simulink model "hexsim_block_model"  (R2015b)
settings: Solver=ode45  StartTime=0.0  StopTime=inf  FixedStep=0.002  RelTol=1e-3
InitFcn:
  | param
values from neighbouring files (symbols this model uses):
  colors = lines(length(row))    [adaptive_coefficients_figure.m]    (also in drawAircraft.m = [edgecolor; edgecolor; edgecolor; edgecolor; footprintcolor])
  V = V*R    [drawAircraft.m]
undefined symbols (not defined in the file or in its folder): attitude_controller, drawAircraft, F, P, position_controller
libraries: simulink x4
settings Model: Creator=beard  LastModifiedBy=magiccjae
settings DataIOCC: SaveFormat=Array  SignalLoggingSaveFormat=ModelDataLogs
settings OptimizationCC: ExpressionDepthLimit=2147483647  InitFltsAndDblsToZero=on
settings DebuggingCC: UnderspecifiedInitializationDetection=Classic  MergeDetectMultiDrivingBlocksExec=none  SolverPrmCheckMsg=warning  FcnCallInpInsideContextMsg=UseLocalSettings  StateNameClashWarn=warning
settings HardwareCC: ProdBitPerPointer=32  ProdLargestAtomicFloat=None  ProdIntDivRoundTo=Undefined  ProdEndianess=Unspecified  ProdWordSize=32  ProdHWDeviceType=32-bit Generic
settings GRTTargetCC: GeneratePreprocessorConditionals=Disable all  CombineOutputUpdateFcns=off  GRTInterface=on
settings ConfigComp: CovModelRefEnable=Off

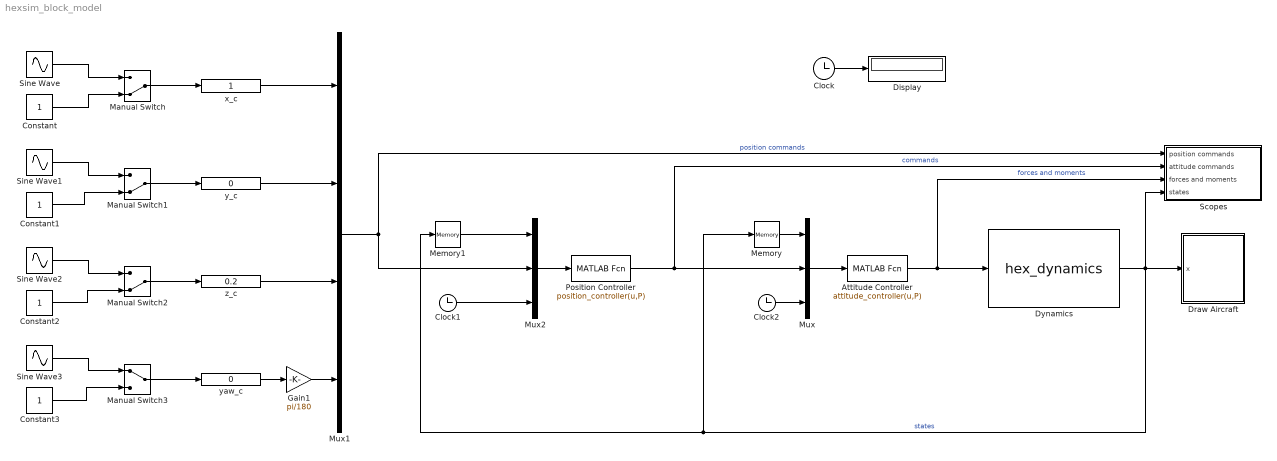
== system hexsim_block_model ==
  Attitude Controller : MATLABFcn  MATLABFcn=attitude_controller(u,P)  OutputDimensions=4  SampleTime=0.002
  Clock : Clock
  Clock1 : Clock
  Clock2 : Clock
  Constant{,1..3} (4 alike) : Constant
  Display : Display
  Draw Aircraft : Subsystem
      mask Display: image(imread('images/tv.jpg'))
  Dynamics : S-Function  FunctionName=hex_dynamics  Parameters=P  SFunctionDeploymentMode=off  EnableBusSupport=off
      mask Display: image(imread('images/hexacopter.png'))
  Gain1 : Gain  Gain=pi/180
  Manual Switch : ManualSwitch  CurrentSetting=0
  Manual Switch1 : ManualSwitch  CurrentSetting=0
  Manual Switch2 : ManualSwitch  CurrentSetting=0
  Manual Switch3 : ManualSwitch
  Memory : Memory
  Memory1 : Memory
  Mux : Mux  Inputs=3
  Mux1 : Mux
  Mux2 : Mux  Inputs=3
  Position Controller : MATLABFcn  MATLABFcn=position_controller(u,P)  OutputDimensions=4  SampleTime=0.01
  Scopes : Subsystem
      mask Display: image(imread('images/scope.jpg'))
  Sine Wave : Sin  Frequency=0.5  Phase=pi/2  SampleTime=0
  Sine Wave1 : Sin  SampleTime=0
  Sine Wave2 : Sin  Amplitude=2  SampleTime=0
  Sine Wave3 : Sin  Amplitude=180  Frequency=0.1  SampleTime=0
  x_c : simulink/Math Operations/Slider Gain  low=-1  gain=1  high=4
  y_c : simulink/Math Operations/Slider Gain  low=-1  gain=0  high=2
  yaw_c : simulink/Math Operations/Slider Gain  low=-180  gain=0  high=180
  z_c : simulink/Math Operations/Slider Gain  low=-5  gain=0.2  high=5
  wires:
  Clock/1 -> Display/1
  y_c/1 -> Mux1/2
  x_c/1 -> Mux1/1
  z_c/1 -> Mux1/3
  yaw_c/1 -> Gain1/1
  Gain1/1 -> Mux1/4
  Manual Switch3/1 -> yaw_c/1
  Manual Switch2/1 -> z_c/1
  Manual Switch1/1 -> y_c/1
  Manual Switch/1 -> x_c/1
  Sine Wave/1 -> Manual Switch/1
  Constant/1 -> Manual Switch/2
  Sine Wave1/1 -> Manual Switch1/1
  Constant1/1 -> Manual Switch1/2
  Sine Wave2/1 -> Manual Switch2/1
  Constant2/1 -> Manual Switch2/2
  Sine Wave3/1 -> Manual Switch3/1
  Constant3/1 -> Manual Switch3/2
  Dynamics/1 -> Memory/1, Memory1/1, Scopes/4(states), Draw Aircraft/1(x)  "states"
  Mux1/1 -> Mux2/2, Scopes/1(position commands)  "position commands"
  Attitude Controller/1 -> Dynamics/1, Scopes/3(forces and moments)  "forces and moments"
  Position Controller/1 -> Mux/2, Scopes/2(attitude commands)  "commands"
  Memory/1 -> Mux/1
  Clock2/1 -> Mux/3
  Mux/1 -> Attitude Controller/1
  Clock1/1 -> Mux2/3
  Mux2/1 -> Position Controller/1
  Memory1/1 -> Mux2/1

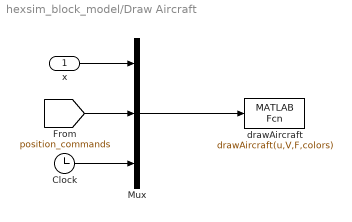
== system hexsim_block_model/Draw Aircraft ==
  x : Inport
  Clock : Clock
  Mux : Mux  Inputs=3
  drawAircraft : MATLABFcn  MATLABFcn=drawAircraft(u,V,F,colors)  OutputDimensions=0  SampleTime=0.1
  wires:
  x/1 -> Mux/1
  Mux/1 -> drawAircraft/1
  [position_commands] -> Mux/2
  Clock/1 -> Mux/3

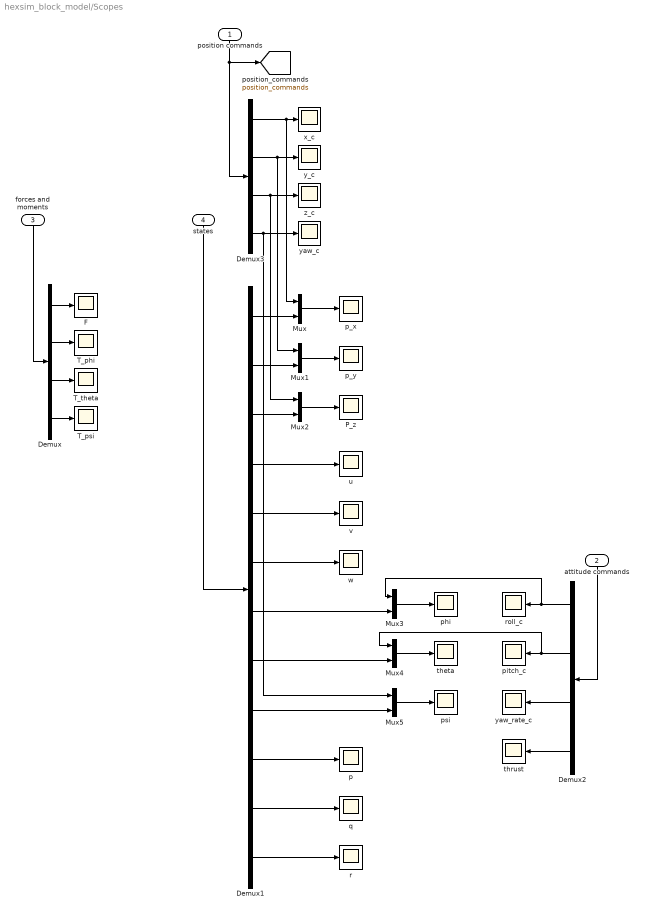
== system hexsim_block_model/Scopes ==
  position commands : Inport
  attitude commands : Inport  Port=2
  forces and moments : Inport  Port=3
  states : Inport  Port=4
  Demux : Demux
  Demux1 : Demux  Outputs=12
  Demux2 : Demux
  Demux3 : Demux
  F : Scope
  Mux{,1..5} (6 alike) : Mux  Inputs=2
  P_z : Scope
  T_phi : Scope
  T_psi : Scope
  T_theta : Scope
  p : Scope
  p_x : Scope
  p_y : Scope
  phi : Scope
  pitch_c : Scope
  psi : Scope
  q : Scope
  r : Scope
  roll_c : Scope
  theta : Scope
  thrust : Scope
  u : Scope
  v : Scope
  w : Scope
  x_c : Scope
  y_c : Scope
  yaw_c : Scope
  yaw_rate_c : Scope
  z_c : Scope
  tag scope: position_commands=global
  wires:
  states/1 -> Demux1/1
  attitude commands/1 -> Demux2/1
  forces and moments/1 -> Demux/1
  Demux/1 -> F/1
  Demux/4 -> T_psi/1
  Demux/2 -> T_phi/1
  Demux/3 -> T_theta/1
  Demux2/4 -> thrust/1
  Demux2/2 -> Mux4/1, pitch_c/1
  Demux2/3 -> yaw_rate_c/1
  position commands/1 -> [position_commands], Demux3/1
  Demux3/1 -> Mux/1, x_c/1
  Demux3/4 -> Mux5/1, yaw_c/1
  Demux3/2 -> Mux1/1, y_c/1
  Demux3/3 -> Mux2/1, z_c/1
  Mux/1 -> p_x/1
  Demux1/1 -> Mux/2
  Demux1/2 -> Mux1/2
  Demux1/3 -> Mux2/2
  Mux1/1 -> p_y/1
  Mux2/1 -> P_z/1
  Mux3/1 -> phi/1
  Mux4/1 -> theta/1
  Mux5/1 -> psi/1
  Demux1/4 -> u/1
  Demux1/5 -> v/1
  Demux1/6 -> w/1
  Demux1/10 -> p/1
  Demux1/11 -> q/1
  Demux1/12 -> r/1
  Demux1/9 -> Mux5/2
  Demux1/8 -> Mux4/2
  Demux1/7 -> Mux3/2
  Demux2/1 -> Mux3/1, roll_c/1
